simulink model "SpringMassDamperSystem"  (R2024a)
settings: Solver=ode45  StartTime=0.0  StopTime=10.0  RelTol=1e-10
settings Model: Creator=tsarg  LastModifiedBy=tsarg

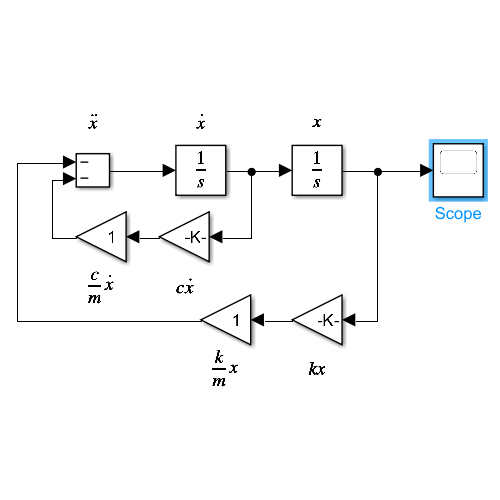
[thumbnail: Simulink's stored preview of the top-level diagram]
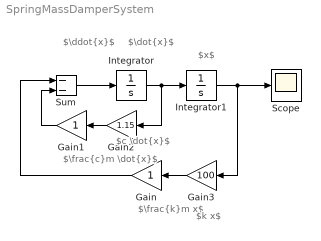
== system SpringMassDamperSystem ==
  note: $\frac{c}m \dot{x}$
  note: $\ddot{x}$
  note: $\dot{x}$
  note: $x$
  note: $\frac{k}m x$
  note: $c \dot{x}$
  note: $k x$
  Gain : Gain
  Gain1 : Gain
  Gain2 : Gain  Gain=1.15
  Gain3 : Gain  Gain=100
  Integrator : Integrator  InitialCondition=1
  Integrator1 : Integrator  InitialCondition=4.5
  Scope : Scope
  Sum : Sum  Inputs=--
  wires:
  Integrator/1 -> Gain2/1, Integrator1/1
  Sum/1 -> Integrator/1
  Integrator1/1 -> Gain3/1, Scope/1
  Gain1/1 -> Sum/2
  Gain/1 -> Sum/1
  Gain2/1 -> Gain1/1
  Gain3/1 -> Gain/1
